simulink model "lab4sim"  (R2022b)
settings: Solver=VariableStepAuto  StartTime=0.0  StopTime=10.0  RelTol=1e-3
values from neighbouring files (symbols this model uses):
  BASE = 11.5 / 100    (= 0.115)    [lab.m]
  goal_x = TARGETS(i, 1)    [lab.m]
  goal_y = TARGETS(i, 2)    [lab.m]
  ini_x = x_out(end)    [lab.m]
  ini_y = y_out(end)    [lab.m]
  J = i^2 * m * r^2 / 2    (= 0.00236430724608)    [lab.m]
  k_e = 0.3953    [lab.m]
  k_m = k_e    (= 0.3953)    [lab.m]
  KR = 30    [lab.m]
  KS = 15    [lab.m]
  L = 0.0047    [lab.m]
  R = 4.8776    [lab.m]
  WHEEL_RADIUS = (7/2) / 100    (= 0.035)    [lab.m]
settings Model: Creator=skifp  LastModifiedBy=skifp

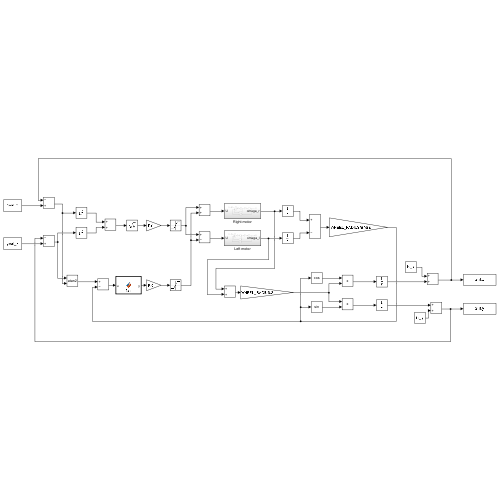
[thumbnail: Simulink's stored preview of the top-level diagram]
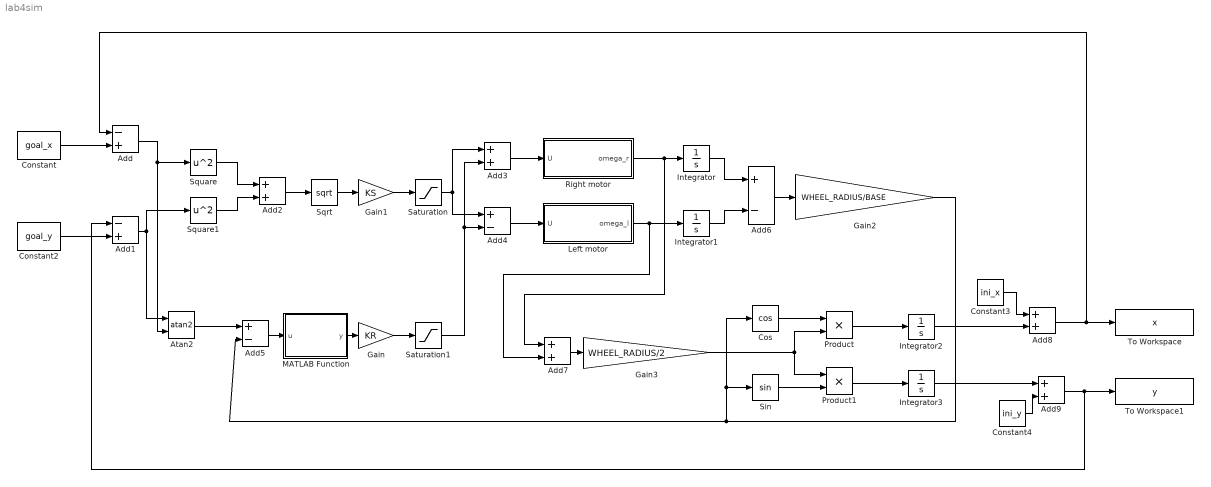
== system lab4sim ==
  Add : Sum  Inputs=-+
  Add1 : Sum  Inputs=-+
  Add{2..3,7..9} (5 alike) : Sum
  Add4 : Sum  Inputs=+-
  Add5 : Sum  Inputs=+-
  Add6 : Sum  Inputs=+-
  Atan2 : Trigonometry  Operator=atan2
  Constant : Constant  Value=goal_x
  Constant2 : Constant  Value=goal_y
  Constant3 : Constant  Value=ini_x
  Constant4 : Constant  Value=ini_y
  Cos : Trigonometry  Operator=cos
  Gain : Gain  Gain=KR
  Gain1 : Gain  Gain=KS
  Gain2 : Gain  Gain=WHEEL_RADIUS/BASE
  Gain3 : Gain  Gain=WHEEL_RADIUS/2
  Integrator{,1..3} (4 alike) : Integrator
  Left motor : Subsystem
  MATLAB Function : MATLAB Function  TreatAsAtomicUnit=on
  Product : Product
  Product1 : Product
  Right motor : Subsystem
  Saturation : Saturate  UpperLimit=80  LowerLimit=-80
  Saturation1 : Saturate  UpperLimit=80  LowerLimit=-80
  Sin : Trigonometry
  Sqrt : Sqrt
  Square : Math  Operator=square
  Square1 : Math  Operator=square
  To Workspace : ToWorkspace  VariableName=x  SaveFormat=Timeseries  SampleTime=-1
  To Workspace1 : ToWorkspace  VariableName=y  SaveFormat=Timeseries  SampleTime=-1
  wires:
  Add/1 -> Square/1, Atan2/2
  Add1/1 -> Square1/1, Atan2/1
  Constant/1 -> Add/2
  Square/1 -> Add2/1
  Square1/1 -> Add2/2
  Add2/1 -> Sqrt/1
  Saturation/1 -> Add4/1, Add3/1
  Atan2/1 -> Add5/1
  Add5/1 -> MATLAB Function/1(u)
  MATLAB Function/1(y) -> Gain/1
  Gain/1 -> Saturation1/1
  Saturation1/1 -> Add4/2, Add3/2
  Sqrt/1 -> Gain1/1
  Gain1/1 -> Saturation/1
  Add3/1 -> Right motor/1(U)
  Add4/1 -> Left motor/1(U)
  Left motor/1(omega_l) -> Integrator1/1, Add7/2
  Right motor/1(omega_r) -> Integrator/1, Add7/1
  Integrator/1 -> Add6/1
  Integrator1/1 -> Add6/2
  Add6/1 -> Gain2/1
  Add7/1 -> Gain3/1
  Gain3/1 -> Product/2, Product1/1
  Cos/1 -> Product/1
  Sin/1 -> Product1/2
  Product/1 -> Integrator2/1
  Product1/1 -> Integrator3/1
  Integrator3/1 -> Add9/1
  Integrator2/1 -> Add8/2
  Constant2/1 -> Add1/2
  Constant3/1 -> Add8/1
  Constant4/1 -> Add9/2
  Gain2/1 -> Add5/2, Sin/1, Cos/1
  Add8/1 -> Add/1, To Workspace/1
  Add9/1 -> Add1/1, To Workspace1/1

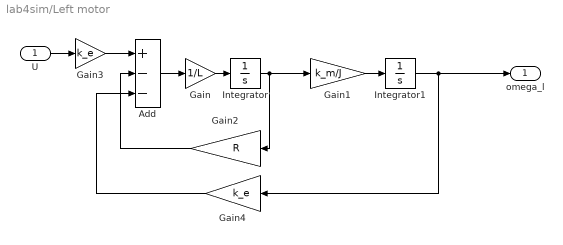
== system lab4sim/Left motor ==
  U : Inport
  Add : Sum  Inputs=+--
  Gain : Gain  Gain=1/L
  Gain1 : Gain  Gain=k_m/J
  Gain2 : Gain  Gain=R
  Gain3 : Gain  Gain=k_e
  Gain4 : Gain  Gain=k_e
  Integrator : Integrator
  Integrator1 : Integrator
  omega_l : Outport
  wires:
  Add/1 -> Gain/1
  Gain4/1 -> Add/3
  Gain1/1 -> Integrator1/1
  Gain/1 -> Integrator/1
  Integrator1/1 -> omega_l/1, Gain4/1
  Integrator/1 -> Gain1/1, Gain2/1
  Gain2/1 -> Add/2
  U/1 -> Gain3/1
  Gain3/1 -> Add/1

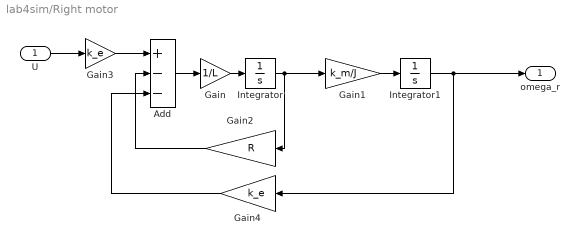
== system lab4sim/Right motor ==
  U : Inport
  Add : Sum  Inputs=+--
  Gain : Gain  Gain=1/L
  Gain1 : Gain  Gain=k_m/J
  Gain2 : Gain  Gain=R
  Gain3 : Gain  Gain=k_e
  Gain4 : Gain  Gain=k_e
  Integrator : Integrator
  Integrator1 : Integrator
  omega_r : Outport
  wires:
  Add/1 -> Gain/1
  Gain4/1 -> Add/3
  Gain1/1 -> Integrator1/1
  Gain/1 -> Integrator/1
  Integrator1/1 -> omega_r/1, Gain4/1
  Integrator/1 -> Gain1/1, Gain2/1
  Gain2/1 -> Add/2
  Gain3/1 -> Add/1
  U/1 -> Gain3/1

== matlab function lab4sim/MATLAB Function ==
  data: u input; y output
function y = fcn(u)

if (u <= -pi)
    y = u + 2*pi;
elseif (u >= pi)
    y = u - 2*pi;
else
    y = u;
end
